simulink model "ProyectoAutomatasSimulink_jona"  (R2017a)
settings: Solver=FixedStepAuto  StartTime=0.0  StopTime=inf  FixedStep=dt  RelTol=1e-3
values from neighbouring files (symbols this model uses):
  amaxh = 1    [ProyectoAutomatas.m]
  amaxt = 1    [ProyectoAutomatas.m]
  bah = Jh*nh*wposh    (= 1200355.55556)    [ProyectoAutomatas.m]
  bat = Jt*nt*wpost    (= 1966933.33333)    [ProyectoAutomatas.m]
  bh = beqh/Rd^2    (= 32)    [ProyectoAutomatas.m]
  bt = beqc/Rw^2    (= 120)    [ProyectoAutomatas.m]
  bw = 30*10^3    (= 30000)    [ProyectoAutomatas.m]
  distanciaSegMaxCarro = geometria.xt_max-constSegCarro    [ProyectoAutomatas.m]
  distanciaSegMinCarro = geometria.xt_min+constSegCarro    [ProyectoAutomatas.m]
  dt = 0.001    [ProyectoAutomatas.m]
  g = 9.80665    [ProyectoAutomatas.m]
  Kisah = Ksah*wposh/nh    (= 150044444444)    [ProyectoAutomatas.m]
  Kisat = Ksat*wpost/nt    (= 245866666667)    [ProyectoAutomatas.m]
  Ksah = bah*wposh    (= 600177777.778)    [ProyectoAutomatas.m]
  Ksat = bat*wpost    (= 983466666.667)    [ProyectoAutomatas.m]
  Kw = 1800*10^3    (= 1800000)    [ProyectoAutomatas.m]
  l_max_cable = 65    [ProyectoAutomatas.m]
  l_min_cable = 5    [ProyectoAutomatas.m]
  lh0 = 5    [ProyectoAutomatas.m]
  longitudSegMaxCable = l_max_cable-constSegCable    (= 60)    [ProyectoAutomatas.m]
  longitudSegMinCable = l_min_cable+constSegCable    (= 10)    [ProyectoAutomatas.m]
  mc = 50000    [ProyectoAutomatas.m]
  Mh = (Jdh+Jmh*rh^2)/Rd^2    (= 48014.2222222)    [ProyectoAutomatas.m]
  ml0 = 15000    [ProyectoAutomatas.m]
  mlfull = 65000    [ProyectoAutomatas.m]
  Mt = mc+(Jwc+Jmc*rc^2)/Rw^2    (= 59008)    [ProyectoAutomatas.m]
  na = 3    [ProyectoAutomatas.m]
  ponderaPIDangulo = -1/1.3e19    (= -7.69230769231e-20)    [ProyectoAutomatas.m]
  rc = 15    [ProyectoAutomatas.m]
  Rd = 0.75    [ProyectoAutomatas.m]
  rh = 30    [ProyectoAutomatas.m]
  Rw = 0.5    [ProyectoAutomatas.m]
  tiempoTransicionAutMan = 1    [ProyectoAutomatas.m]
  vh0 = 0    [ProyectoAutomatas.m]
  vlx0 = 0    [ProyectoAutomatas.m]
  vly0 = 0    [ProyectoAutomatas.m]
  vmaxh = 3    [ProyectoAutomatas.m]
  vmaxhfull = 1.5    [ProyectoAutomatas.m]
  vmaxhSobrepeso = 0.1    [ProyectoAutomatas.m]
  vmaxt = 4    [ProyectoAutomatas.m]
  vt0 = 0    [ProyectoAutomatas.m]
  xl0 = -30    [ProyectoAutomatas.m]
  xt0 = -30    [ProyectoAutomatas.m]
  xt_max = 50    [ProyectoAutomatas.m]
  xt_max_max = 51    [ProyectoAutomatas.m]
  xt_min = -30    [ProyectoAutomatas.m]
  yl0 = yt0-lh0-ml0*g/Kw    (= 39.9182779167)    [ProyectoAutomatas.m]
  yt0 = 45    [ProyectoAutomatas.m]
undefined symbols (not defined in the file or in its folder): geometria
libraries: vrlib x1
settings Model: Creator=Garcia Obredor  LastModifiedBy=yellow submarine
settings DataIOCC: LimitDataPoints=on  SaveFormat=Array  SignalLoggingSaveFormat=ModelDataLogs
settings OptimizationCC: BlockReduction=off  BooleanDataType=off  LifeSpan=inf
settings DebuggingCC: SaveWithParameterizedLinksMsg=none  UnderspecifiedInitializationDetection=Classic  MergeDetectMultiDrivingBlocksExec=none  SignalResolutionControl=TryResolveAllWithWarning  MultiTaskDSMMsg=warning  MultiTaskCondExecSysMsg=none  SFUnexpectedBacktrackingDiag=warning  SFNoUnconditionalDefaultTransitionDiag=warning  SFExecutionAtInitializationDiag=none
settings HardwareCC: ProdBitPerPointer=32  ProdBitPerSizeT=32  ProdBitPerPtrDiffT=32  ProdLargestAtomicFloat=None  ProdIntDivRoundTo=Undefined  ProdEndianess=Unspecified  ProdWordSize=32  ProdHWDeviceType=32-bit Generic  TargetBitPerPointer=64  TargetBitPerSizeT=64  TargetBitPerPtrDiffT=64  TargetLongLongMode=on  TargetIntDivRoundTo=Zero  TargetEndianess=LittleEndian  TargetWordSize=64  TargetHWDeviceType=MATLAB Host  ProdEqTarget=off
settings ModelReferenceCC: PropagateSignalLabelsOutOfModel=off
settings GRTTargetCC: TargetLangStandard=C89/C90 (ANSI)  GeneratePreprocessorConditionals=Disable all
settings ConfigComp: CovMetricSettings=dw  CovHtmlReporting=on  CovSaveCumulativeToWorkspaceVar=on  CovSaveSingleToWorkspaceVar=on  CovExternalEMLEnable=off

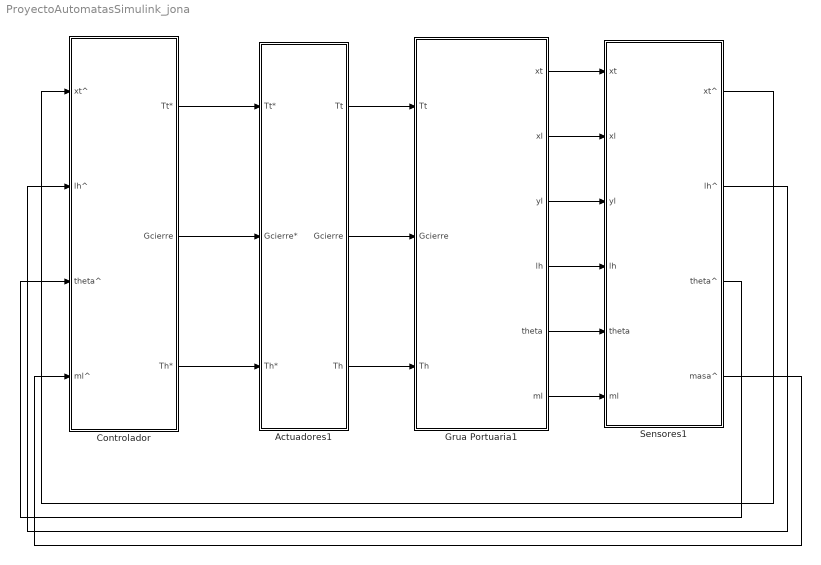
== system ProyectoAutomatasSimulink_jona ==
  Actuadores1 : Subsystem
  Controlador : Subsystem
  Grua Portuaria1 : Subsystem
  Sensores1 : Subsystem
  wires:
  Controlador/2(Gcierre) -> Actuadores1/2(Gcierre*)
  Grua Portuaria1/6(ml) -> Sensores1/6(ml)
  Grua Portuaria1/1(xt) -> Sensores1/1(xt)
  Actuadores1/2(Gcierre) -> Grua Portuaria1/2(Gcierre)
  Grua Portuaria1/5(theta) -> Sensores1/5(theta)
  Controlador/3(Th*) -> Actuadores1/3(Th*)
  Actuadores1/3(Th) -> Grua Portuaria1/3(Th)
  Actuadores1/1(Tt) -> Grua Portuaria1/1(Tt)
  Grua Portuaria1/3(yl) -> Sensores1/3(yl)
  Grua Portuaria1/4(lh) -> Sensores1/4(lh)
  Controlador/1(Tt*) -> Actuadores1/1(Tt*)
  Grua Portuaria1/2(xl) -> Sensores1/2(xl)
  Sensores1/1(xt^) -> Controlador/1(xt^)
  Sensores1/2(lh^) -> Controlador/2(lh^)
  Sensores1/3(theta^) -> Controlador/3(theta^)
  Sensores1/4(masa^) -> Controlador/4(ml^)

== system ProyectoAutomatasSimulink_jona/Actuadores1 ==
  Tt* : Inport
  Gcierre* : Inport  Port=2
  Th* : Inport  Port=3
  Tt : Outport
  Gcierre : Outport  Port=2
  Th : Outport  Port=3
  wires:
  Tt*/1 -> Tt/1  "Tt"
  Th*/1 -> Th/1  "Th"
  Gcierre*/1 -> Gcierre/1

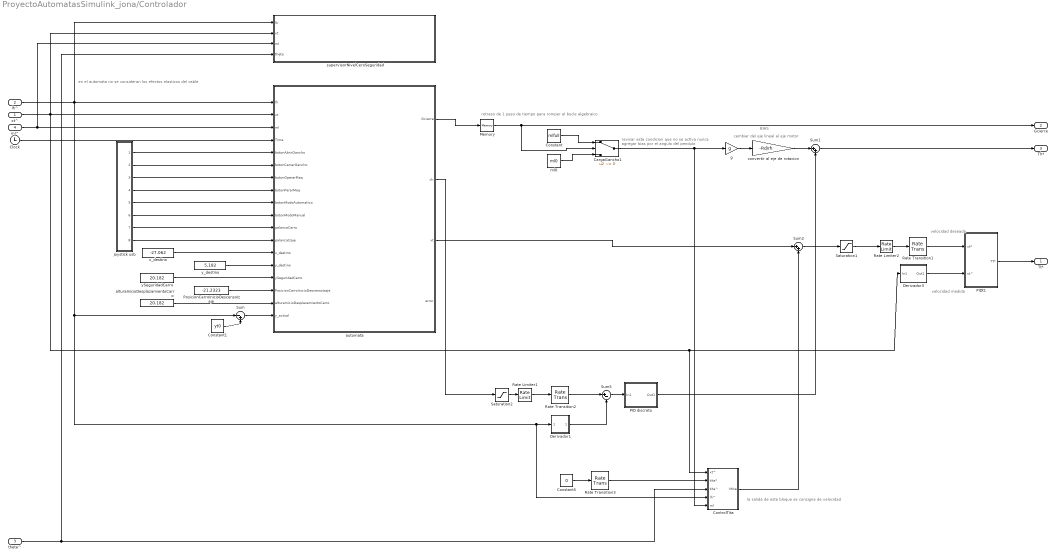
== system ProyectoAutomatasSimulink_jona/Controlador ==
  note: la salida de este bloque es consigna de velocidad
  note: cambiar del eje lineal al eje motor
  note: revisar esta condicion que no se activa nunca
      | agregar bias por el angulo del pendulo
  note: BIAS
  note: velocidad medida
  note: velocidad deseada
  note: retraso de 1 paso de tiempo para romper el bucle algebraico
  note: en el automata no se consideran los efectos elasticos del cable
  xt^ : Inport
  lh^ : Inport  Port=2
  theta^ : Inport  Port=3
  ml^ : Inport  Port=4
  CargaGancho1 : Switch  Criteria=u2 ~= 0  Threshold=0.5
  Clock : Clock
  Constant : Constant  Value=mlfull
  Constant1 : Constant  Value=yt0
  Constant5 : Constant  Value=0
  ControlTita : Subsystem
  Derivador1 : Subsystem
  Derivador3 : Subsystem
  Memory : Memory
  PID discreto : Subsystem
  PIDt1 : Subsystem
  PosicionCarroInicioDescensoIzaje : Constant  Value=-21.2323
  Rate Limiter1 : RateLimiter  RisingSlewLimit=amaxh  FallingSlewLimit=-amaxh  SampleTimeMode=inherited
  Rate Limiter2 : RateLimiter  RisingSlewLimit=amaxt  FallingSlewLimit=-amaxt  SampleTimeMode=inherited
  Rate Transition1 : RateTransition  OutPortSampleTime=dt
  Rate Transition2 : RateTransition  X0=5  OutPortSampleTime=dt
  Rate Transition3 : RateTransition  OutPortSampleTime=dt
  Saturation1 : Saturate  UpperLimit=vmaxt  LowerLimit=-vmaxt
  Saturation2 : Saturate  UpperLimit=vmaxh  LowerLimit=-vmaxh
  Sum : Sum  Inputs=|-+
  Sum1 : Sum  Inputs=|++
  Sum2 : Sum  Inputs=|++
  Sum5 : Sum  Inputs=|+-
  alturaInicioDesplazamientoCarro : Constant  Value=20.182
  automata : Stateflow chart  TreatAsAtomicUnit=on
  convertir al eje de rotacion : Gain  Gain=-Rd/rh
  g : Gain  Gain=g
  joystick usb : Subsystem
  "ml0 " : Constant  Value=ml0
  supervisorNivelCeroSeguridad : Stateflow chart  TreatAsAtomicUnit=on
  x_destino : Constant  Value=-27.062
  ySeguridadCarro : Constant  Value=20.182
  y_destino : Constant  Value=5.182
  Tt* : Outport
  Gcierre : Outport  Port=2
  Th* : Outport  Port=3
  wires:
  ml^/1 -> automata/3(ml), supervisorNivelCeroSeguridad/3(ml)
  automata/2(vh) -> Saturation2/1
  joystick usb/7(Out8) -> automata/11(palancaCarro)
  joystick usb/1(Out1) -> automata/5(botonAbrirGancho)
  joystick usb/2(Out2) -> automata/6(botonCerrarGancho)
  joystick usb/8(Out9) -> automata/12(palancaIzaje)
  joystick usb/4(Out4) -> automata/8(botonPararMaq)
  joystick usb/5(Out6) -> automata/9(botonModoAutomatico)
  joystick usb/6(Out7) -> automata/10(botonModoManual)
  joystick usb/3(Out3) -> automata/7(botonOperarMaq)
  Saturation1/1 -> Rate Limiter2/1
  Rate Transition1/1 -> PIDt1/1(xt*)
  Rate Limiter2/1 -> Rate Transition1/1
  Derivador3/1(Out1) -> PIDt1/2(xt^)
  xt^/1 -> supervisorNivelCeroSeguridad/2(xt), automata/2(xt), Derivador3/1(In1), ControlTita/1(xt^)
  Sum1/1 -> Th*/1
  automata/1(Gcierre) -> Memory/1
  "ml0 "/1 -> CargaGancho1/3
  Constant/1 -> CargaGancho1/1
  Memory/1 -> CargaGancho1/2, Gcierre/1
  PIDt1/1(Tt*) -> Tt*/1
  g/1 -> convertir al eje de rotacion/1
  convertir al eje de rotacion/1 -> Sum1/1
  PID discreto/1(Out1) -> Sum1/2
  Rate Transition2/1 -> Sum5/1
  Sum5/1 -> PID discreto/1(In1)
  Rate Limiter1/1 -> Rate Transition2/1
  Saturation2/1 -> Rate Limiter1/1
  Derivador1/1(Out1) -> Sum5/2
  automata/3(vt) -> Sum2/1
  Constant5/1 -> Rate Transition3/1
  Rate Transition3/1 -> ControlTita/2(tita*)
  lh^/1 -> supervisorNivelCeroSeguridad/1(lh), automata/1(lh), ControlTita/4(lh^), Derivador1/1(In1), Sum/1
  theta^/1 -> ControlTita/3(tita^), supervisorNivelCeroSeguridad/4(theta)
  CargaGancho1/1 -> ControlTita/5(ml), g/1
  ySeguridadCarro/1 -> automata/15(ySeguridadCarro)
  PosicionCarroInicioDescensoIzaje/1 -> automata/16(PosicionCarroInicioDescensoIzaje)
  alturaInicioDesplazamientoCarro/1 -> automata/17(alturaInicioDesplazamientoCarro)
  x_destino/1 -> automata/13(x_destino)
  Constant1/1 -> Sum/2
  Sum/1 -> automata/18(y_actual)
  y_destino/1 -> automata/14(y_destino)
  Sum2/1 -> Saturation1/1
  ControlTita/1(Vtita) -> Sum2/2
  Clock/1 -> automata/4(Time)

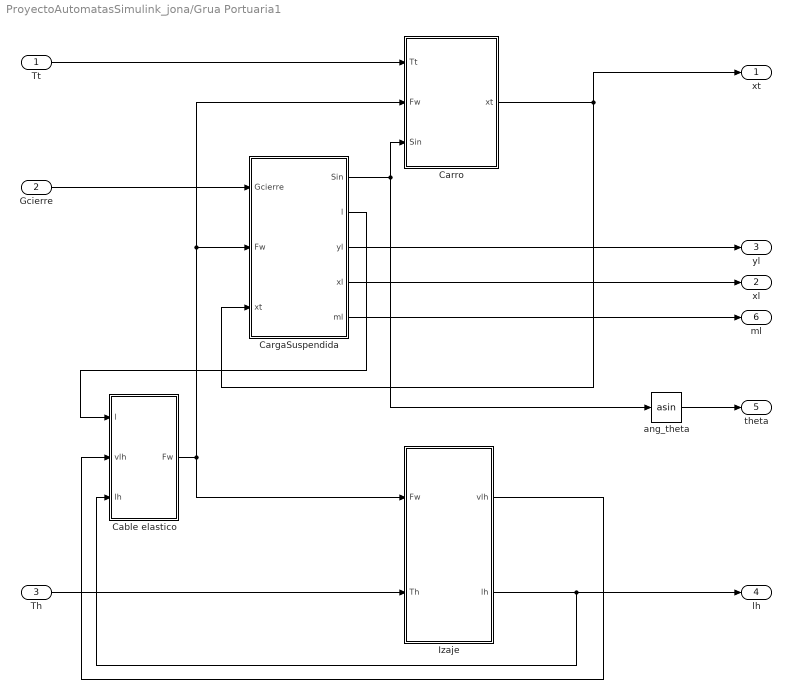
== system ProyectoAutomatasSimulink_jona/Grua Portuaria1 ==
  Tt : Inport
  Gcierre : Inport  Port=2
  Th : Inport  Port=3
  Cable elastico : Subsystem
  CargaSuspendida : Subsystem
  Carro : Subsystem
  Izaje : Subsystem
  ang_theta : Trigonometry  Operator=asin
  xt : Outport
  xl : Outport  Port=2
  yl : Outport  Port=3
  lh : Outport  Port=4
  theta : Outport  Port=5
  ml : Outport  Port=6
  wires:
  Izaje/1(vlh) -> Cable elastico/2(vlh)
  CargaSuspendida/1(Sin) -> Carro/3(Sin), ang_theta/1
  Th/1 -> Izaje/2(Th)
  Izaje/2(lh) -> Cable elastico/3(lh), lh/1
  Carro/1(xt) -> xt/1, CargaSuspendida/3(xt)
  Gcierre/1 -> CargaSuspendida/1(Gcierre)
  Tt/1 -> Carro/1(Tt)
  CargaSuspendida/2(l) -> Cable elastico/1(l)
  Cable elastico/1(Fw) -> Izaje/1(Fw), Carro/2(Fw), CargaSuspendida/2(Fw)
  ang_theta/1 -> theta/1
  CargaSuspendida/5(ml) -> ml/1
  CargaSuspendida/4(xl) -> xl/1
  CargaSuspendida/3(yl) -> yl/1

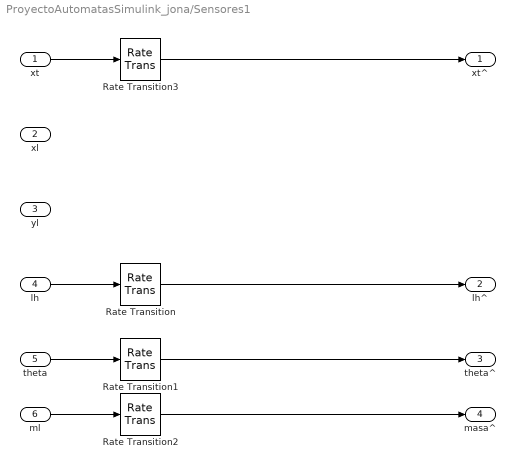
== system ProyectoAutomatasSimulink_jona/Sensores1 ==
  xt : Inport
  xl : Inport  Port=2
  yl : Inport  Port=3
  lh : Inport  Port=4
  theta : Inport  Port=5
  ml : Inport  Port=6
  Rate Transition : RateTransition  X0=5  OutPortSampleTime=dt
  Rate Transition1 : RateTransition  OutPortSampleTime=dt
  Rate Transition2 : RateTransition  X0=ml0  OutPortSampleTime=dt
  Rate Transition3 : RateTransition  X0=-30  OutPortSampleTime=dt
  xt^ : Outport
  lh^ : Outport  Port=2
  theta^ : Outport  Port=3
  masa^ : Outport  Port=4
  wires:
  theta/1 -> Rate Transition1/1
  xt/1 -> Rate Transition3/1
  Rate Transition1/1 -> theta^/1
  ml/1 -> Rate Transition2/1
  lh/1 -> Rate Transition/1
  Rate Transition/1 -> lh^/1
  Rate Transition3/1 -> xt^/1
  Rate Transition2/1 -> masa^/1

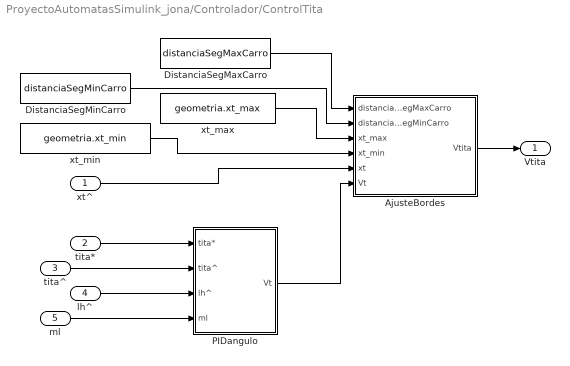
== system ProyectoAutomatasSimulink_jona/Controlador/ControlTita ==
  xt^ : Inport
  tita* : Inport  Port=2
  tita^ : Inport  Port=3
  lh^ : Inport  Port=4
  ml : Inport  Port=5
  AjusteBordes : MATLAB Function  TreatAsAtomicUnit=on
  DistanciaSegMaxCarro : Constant  Value=distanciaSegMaxCarro
  DistanciaSegMinCarro : Constant  Value=distanciaSegMinCarro
  PIDangulo : Subsystem
  xt_max : Constant  Value=geometria.xt_max
  xt_min : Constant  Value=geometria.xt_min
  Vtita : Outport
  wires:
  tita*/1 -> PIDangulo/1(tita*)
  ml/1 -> PIDangulo/4(ml)
  lh^/1 -> PIDangulo/3(lh^)
  AjusteBordes/1(Vtita) -> Vtita/1
  tita^/1 -> PIDangulo/2(tita^)
  PIDangulo/1(Vt) -> AjusteBordes/6(Vt)
  xt^/1 -> AjusteBordes/5(xt)
  DistanciaSegMaxCarro/1 -> AjusteBordes/1(distanciaSegMaxCarro)
  DistanciaSegMinCarro/1 -> AjusteBordes/2(distanciaSegMinCarro)
  xt_max/1 -> AjusteBordes/3(xt_max)
  xt_min/1 -> AjusteBordes/4(xt_min)

== system ProyectoAutomatasSimulink_jona/Controlador/Derivador1 ==
  In1 : Inport
  1/dt : Gain  Gain=1/dt
  Delay3 : Delay  DelayLength=1  InitialCondition=5  SampleTime=dt
  Sum6 : Sum  Inputs=|+-
  Out1 : Outport
  wires:
  In1/1 -> Delay3/1, Sum6/1
  Delay3/1 -> Sum6/2
  Sum6/1 -> 1/dt/1
  1/dt/1 -> Out1/1

== system ProyectoAutomatasSimulink_jona/Controlador/Derivador3 ==
  In1 : Inport
  1/dt : Gain  Gain=1/dt
  Delay3 : Delay  DelayLength=1  InitialCondition=-30  SampleTime=dt
  Sum6 : Sum  Inputs=|+-
  Out1 : Outport
  wires:
  In1/1 -> Delay3/1, Sum6/1
  Delay3/1 -> Sum6/2
  Sum6/1 -> 1/dt/1
  1/dt/1 -> Out1/1

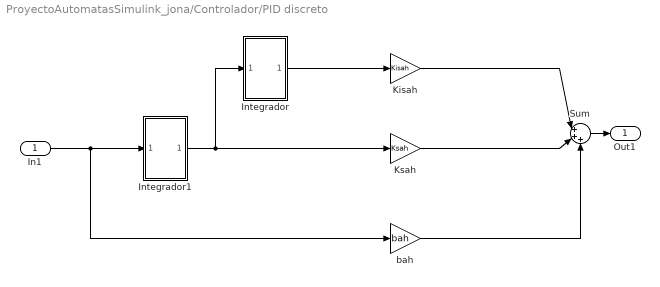
== system ProyectoAutomatasSimulink_jona/Controlador/PID discreto ==
  In1 : Inport
  Integrador : Subsystem
  Integrador1 : Subsystem
  Kisah : Gain  Gain=Kisah
  Ksah : Gain  Gain=Ksah
  Sum : Sum  Inputs=|+++
  bah : Gain  Gain=bah
  Out1 : Outport
  wires:
  In1/1 -> Integrador1/1(In1), bah/1
  bah/1 -> Sum/3
  Sum/1 -> Out1/1
  Ksah/1 -> Sum/2
  Kisah/1 -> Sum/1
  Integrador/1(Out1) -> Kisah/1
  Integrador1/1(Out1) -> Integrador/1(In1), Ksah/1

== system ProyectoAutomatasSimulink_jona/Controlador/PIDt1 ==
  xt* : Inport
  xt^ : Inport  Port=2
  PID discreto : Subsystem
  Scope : Scope
  Sum5 : Sum  Inputs=|+-
  Tt* : Outport
  wires:
  xt*/1 -> Sum5/1
  xt^/1 -> Sum5/2
  Sum5/1 -> Scope/1, PID discreto/1(In1)
  PID discreto/1(Out1) -> Tt*/1

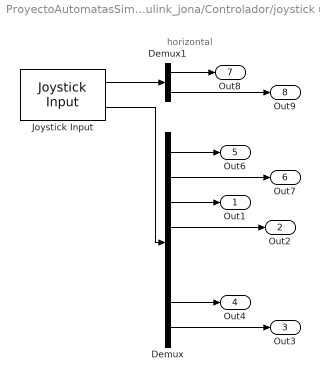
== system ProyectoAutomatasSimulink_jona/Controlador/joystick usb ==
  note: horizontal
  Demux : Demux  Outputs=8
  Demux1 : Demux  Outputs=2
  Joystick Input : vrlib/Joystick Input  joyid=1  adjustports=on  forcefeed=off
      settings: SourceProductBaseCode=VR
  Out1 : Outport
  Out2 : Outport  Port=2
  Out3 : Outport  Port=3
  Out4 : Outport  Port=4
  Out6 : Outport  Port=5
  Out7 : Outport  Port=6
  Out8 : Outport  Port=7
  Out9 : Outport  Port=8
  wires:
  Demux/8 -> Out3/1
  Demux/1 -> Out6/1
  Joystick Input/2 -> Demux/1
  Demux/2 -> Out7/1
  Joystick Input/1 -> Demux1/1
  Demux/7 -> Out4/1
  Demux1/1 -> Out8/1
  Demux1/2 -> Out9/1
  Demux/4 -> Out2/1
  Demux/3 -> Out1/1

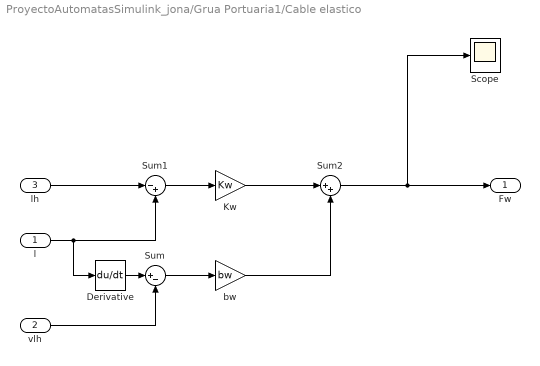
== system ProyectoAutomatasSimulink_jona/Grua Portuaria1/Cable elastico ==
  l : Inport
  vlh : Inport  Port=2
  lh : Inport  Port=3
  Derivative : Derivative
  Kw : Gain  Gain=Kw
  Scope : Scope
  Sum : Sum  Inputs=|+-
  Sum1 : Sum  Inputs=|-+
  Sum2 : Sum  Inputs=|++
  bw : Gain  Gain=bw
  Fw : Outport
  wires:
  l/1 -> Derivative/1, Sum1/2
  Derivative/1 -> Sum/1
  vlh/1 -> Sum/2
  Sum1/1 -> Kw/1
  Sum/1 -> bw/1
  Kw/1 -> Sum2/1
  bw/1 -> Sum2/2
  Sum2/1 -> Scope/1, Fw/1
  lh/1 -> Sum1/1

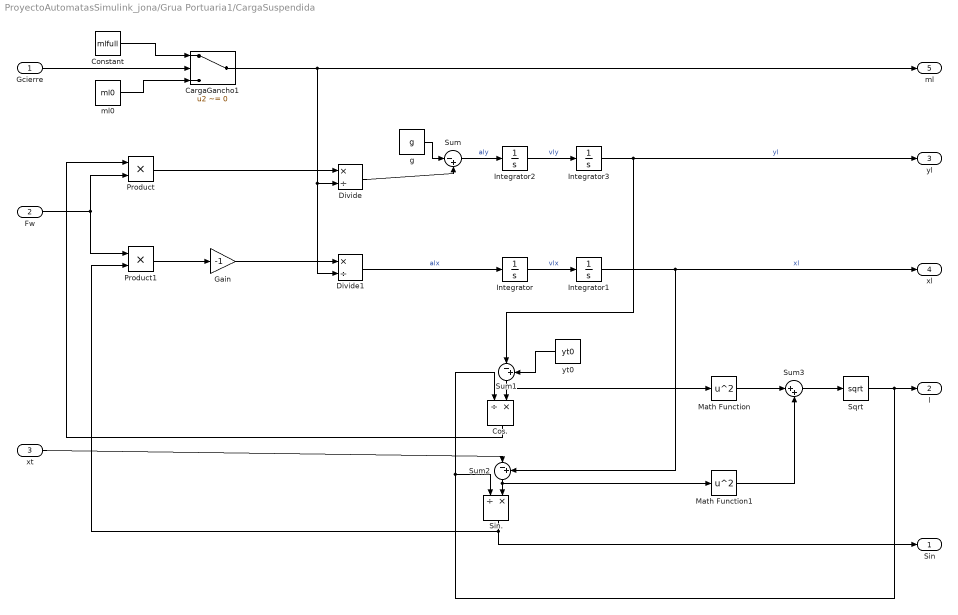
== system ProyectoAutomatasSimulink_jona/Grua Portuaria1/CargaSuspendida ==
  Gcierre : Inport
  Fw : Inport  Port=2
  xt : Inport  Port=3
  CargaGancho1 : Switch  Criteria=u2 ~= 0  Threshold=0.5
  Constant : Constant  Value=mlfull
  Cos. : Product  Inputs=/*
  Divide : Product  Inputs=*/
  Divide1 : Product  Inputs=*/
  Gain : Gain  Gain=-1
  Integrator : Integrator  InitialCondition=vlx0
  Integrator1 : Integrator  InitialCondition=xl0
  Integrator2 : Integrator  InitialCondition=vly0
  Integrator3 : Integrator  InitialCondition=yl0
  Math Function : Math  Operator=square  SaturateOnIntegerOverflow=on
  Math Function1 : Math  Operator=square  SaturateOnIntegerOverflow=on
  Product : Product
  Product1 : Product
  Sin. : Product  Inputs=/*
  Sqrt : Sqrt  SaturateOnIntegerOverflow=on
  Sum : Sum  Inputs=|-+
  Sum1 : Sum  Inputs=|-+
  Sum2 : Sum  Inputs=|-+
  Sum3 : Sum  Inputs=|++
  g : Constant  Value=g
  "ml0 " : Constant  Value=ml0
  yt0 : Constant  Value=yt0
  Sin : Outport
  l : Outport  Port=2
  yl : Outport  Port=3
  xl : Outport  Port=4
  ml : Outport  Port=5
  wires:
  CargaGancho1/1 -> ml/1, Divide/2, Divide1/2
  Gcierre/1 -> CargaGancho1/2
  Fw/1 -> Product1/1, Product/2
  Product/1 -> Divide/1
  Product1/1 -> Gain/1
  Gain/1 -> Divide1/1
  Divide/1 -> Sum/2
  g/1 -> Sum/1
  Integrator/1 -> Integrator1/1  "vlx"
  Integrator1/1 -> xl/1, Sum2/2  "xl"
  Integrator2/1 -> Integrator3/1  "vly"
  Sum1/1 -> Cos./2, Math Function/1
  yt0/1 -> Sum1/2
  Integrator3/1 -> Sum1/1, yl/1  "yl"
  Cos./1 -> Product/1
  Sum2/1 -> Math Function1/1, Sin./2
  xt/1 -> Sum2/1
  Sin./1 -> Sin/1, Product1/2
  Math Function/1 -> Sum3/1
  Math Function1/1 -> Sum3/2
  Sum3/1 -> Sqrt/1
  Constant/1 -> CargaGancho1/1
  "ml0 "/1 -> CargaGancho1/3
  Sqrt/1 -> Cos./1, Sin./1, l/1
  Sum/1 -> Integrator2/1  "aly"
  Divide1/1 -> Integrator/1  "alx"

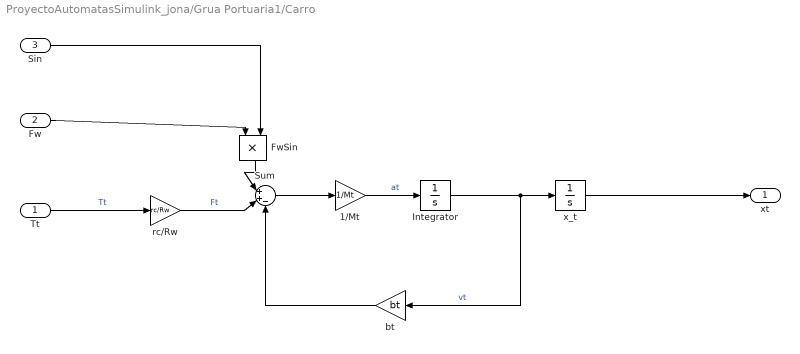
== system ProyectoAutomatasSimulink_jona/Grua Portuaria1/Carro ==
  Tt : Inport
  Fw : Inport  Port=2
  Sin : Inport  Port=3
  1/Mt : Gain  Gain=1/Mt
  FwSin : Product
  Integrator : Integrator  InitialCondition=vt0
  Sum : Sum  Inputs=|++-
  bt : Gain  Gain=bt
  rc/Rw : Gain  Gain=rc/Rw
  x_t : Integrator  InitialCondition=xt0
  xt : Outport
  wires:
  x_t/1 -> xt/1
  rc/Rw/1 -> Sum/2  "Ft"
  Tt/1 -> rc/Rw/1  "Tt"
  1/Mt/1 -> Integrator/1  "at"
  bt/1 -> Sum/3
  Sum/1 -> 1/Mt/1
  Integrator/1 -> bt/1, x_t/1  "vt"
  Sin/1 -> FwSin/2
  FwSin/1 -> Sum/1
  Fw/1 -> FwSin/1

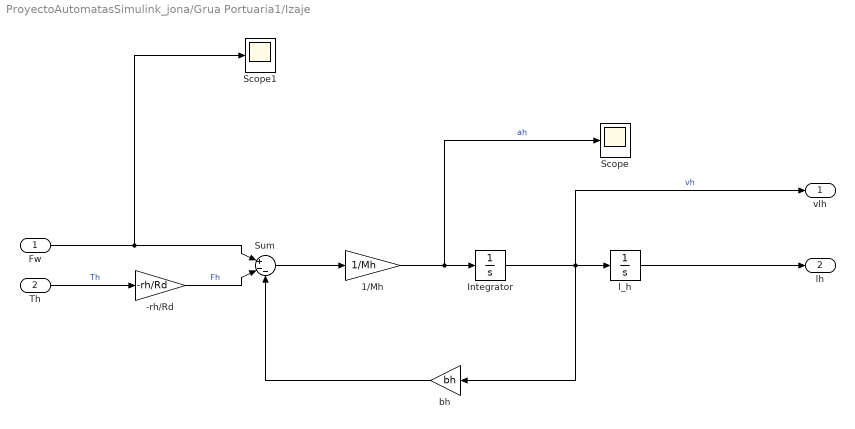
== system ProyectoAutomatasSimulink_jona/Grua Portuaria1/Izaje ==
  Fw : Inport
  Th : Inport  Port=2
  "-rh/Rd\t" : Gain  Gain=-rh/Rd
  1/Mh : Gain  Gain=1/Mh
  Integrator : Integrator  InitialCondition=vh0
  Scope : Scope
  Scope1 : Scope
  Sum : Sum  Inputs=|+--
  bh : Gain  Gain=bh
  l_h : Integrator  InitialCondition=lh0
  vlh : Outport
  lh : Outport  Port=2
  wires:
  l_h/1 -> lh/1
  "-rh/Rd\t"/1 -> Sum/2  "Fh"
  Th/1 -> "-rh/Rd\t"/1  "Th"
  1/Mh/1 -> Scope/1, Integrator/1  "ah"
  bh/1 -> Sum/3
  Sum/1 -> 1/Mh/1
  Integrator/1 -> vlh/1, bh/1, l_h/1  "vh"
  Fw/1 -> Scope1/1, Sum/1

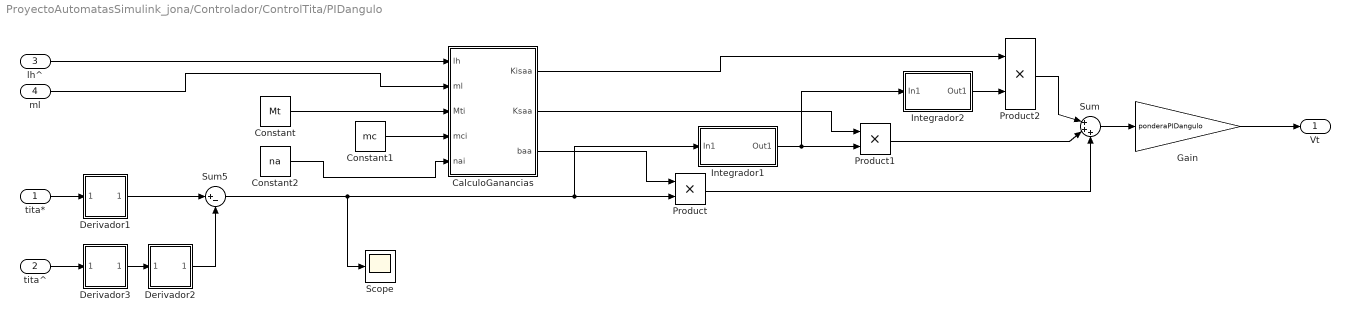
== system ProyectoAutomatasSimulink_jona/Controlador/ControlTita/PIDangulo ==
  tita* : Inport
  tita^ : Inport  Port=2
  lh^ : Inport  Port=3
  ml : Inport  Port=4
  CalculoGanancias : MATLAB Function  TreatAsAtomicUnit=on
  Constant : Constant  Value=Mt
  Constant1 : Constant  Value=mc
  Constant2 : Constant  Value=na
  Derivador1 : Subsystem
  Derivador2 : Subsystem
  Derivador3 : Subsystem
  Gain : Gain  Gain=ponderaPIDangulo
  Integrador1 : Subsystem
  Integrador2 : Subsystem
  Product : Product
  Product1 : Product
  Product2 : Product
  Scope : Scope
  Sum : Sum  Inputs=|+++
  Sum5 : Sum  Inputs=|+-
  Vt : Outport
  wires:
  tita*/1 -> Derivador1/1(In1)
  lh^/1 -> CalculoGanancias/1(lh)
  Sum/1 -> Gain/1
  Product/1 -> Sum/3
  Integrador1/1(Out1) -> Integrador2/1(In1), Product1/2
  Product1/1 -> Sum/2
  Integrador2/1(Out1) -> Product2/2
  tita^/1 -> Derivador3/1(In1)
  Sum5/1 -> Scope/1, Integrador1/1(In1), Product/2
  CalculoGanancias/3(baa) -> Product/1
  CalculoGanancias/2(Ksaa) -> Product1/1
  CalculoGanancias/1(Kisaa) -> Product2/1
  ml/1 -> CalculoGanancias/2(ml)
  Constant/1 -> CalculoGanancias/3(Mti)
  Constant1/1 -> CalculoGanancias/4(mci)
  Constant2/1 -> CalculoGanancias/5(nai)
  Derivador3/1(Out1) -> Derivador2/1(In1)
  Derivador1/1(Out1) -> Sum5/1
  Gain/1 -> Vt/1
  Product2/1 -> Sum/1
  Derivador2/1(Out1) -> Sum5/2

== system ProyectoAutomatasSimulink_jona/Controlador/PID discreto/Integrador ==
  In1 : Inport
  Delay3 : Delay  DelayLength=1  SampleTime=dt
  Sum6 : Sum  Inputs=|++
  dt : Gain  Gain=dt
  Out1 : Outport
  wires:
  Delay3/1 -> Sum6/2
  Sum6/1 -> Out1/1, Delay3/1
  dt/1 -> Sum6/1
  In1/1 -> dt/1

== system ProyectoAutomatasSimulink_jona/Controlador/PID discreto/Integrador1 ==
  In1 : Inport
  Delay3 : Delay  DelayLength=1  SampleTime=dt
  Sum6 : Sum  Inputs=|++
  dt : Gain  Gain=dt
  Out1 : Outport
  wires:
  Delay3/1 -> Sum6/2
  Sum6/1 -> Out1/1, Delay3/1
  dt/1 -> Sum6/1
  In1/1 -> dt/1

== system ProyectoAutomatasSimulink_jona/Controlador/PIDt1/PID discreto ==
  In1 : Inport
  Integrador : Subsystem
  Integrador1 : Subsystem
  Kisat : Gain  Gain=Kisat
  Ksat : Gain  Gain=Ksat
  Sum : Sum  Inputs=|+++
  bat : Gain  Gain=bat
  Out1 : Outport
  wires:
  bat/1 -> Sum/3
  Ksat/1 -> Sum/2
  Kisat/1 -> Sum/1
  Sum/1 -> Out1/1
  In1/1 -> Integrador1/1(In1), bat/1
  Integrador/1(Out1) -> Kisat/1
  Integrador1/1(Out1) -> Integrador/1(In1), Ksat/1

== system ProyectoAutomatasSimulink_jona/Controlador/ControlTita/PIDangulo/Derivador1 ==
  In1 : Inport
  1/dt : Gain  Gain=1/dt
  Delay3 : Delay  DelayLength=1  InitialCondition=0  SampleTime=dt
  Sum6 : Sum  Inputs=|+-
  Out1 : Outport
  wires:
  In1/1 -> Delay3/1, Sum6/1
  Delay3/1 -> Sum6/2
  Sum6/1 -> 1/dt/1
  1/dt/1 -> Out1/1

== system ProyectoAutomatasSimulink_jona/Controlador/ControlTita/PIDangulo/Derivador2 ==
  In1 : Inport
  1/dt : Gain  Gain=1/dt
  Delay3 : Delay  DelayLength=1  InitialCondition=0  SampleTime=dt
  Sum6 : Sum  Inputs=|+-
  Out1 : Outport
  wires:
  In1/1 -> Delay3/1, Sum6/1
  Delay3/1 -> Sum6/2
  Sum6/1 -> 1/dt/1
  1/dt/1 -> Out1/1

== system ProyectoAutomatasSimulink_jona/Controlador/ControlTita/PIDangulo/Derivador3 ==
  In1 : Inport
  1/dt : Gain  Gain=1/dt
  Delay3 : Delay  DelayLength=1  InitialCondition=0  SampleTime=dt
  Sum6 : Sum  Inputs=|+-
  Out1 : Outport
  wires:
  In1/1 -> Delay3/1, Sum6/1
  Delay3/1 -> Sum6/2
  Sum6/1 -> 1/dt/1
  1/dt/1 -> Out1/1

== system ProyectoAutomatasSimulink_jona/Controlador/ControlTita/PIDangulo/Integrador1 ==
  In1 : Inport
  Delay3 : Delay  DelayLength=1  SampleTime=dt
  Sum6 : Sum  Inputs=|++
  dt : Gain  Gain=dt
  Out1 : Outport
  wires:
  Delay3/1 -> Sum6/2
  Sum6/1 -> Out1/1, Delay3/1
  dt/1 -> Sum6/1
  In1/1 -> dt/1

== system ProyectoAutomatasSimulink_jona/Controlador/ControlTita/PIDangulo/Integrador2 ==
  In1 : Inport
  Delay3 : Delay  DelayLength=1  SampleTime=dt
  Sum6 : Sum  Inputs=|++
  dt : Gain  Gain=dt
  Out1 : Outport
  wires:
  Delay3/1 -> Sum6/2
  Sum6/1 -> Out1/1, Delay3/1
  dt/1 -> Sum6/1
  In1/1 -> dt/1

== system ProyectoAutomatasSimulink_jona/Controlador/PIDt1/PID discreto/Integrador ==
  In1 : Inport
  Delay3 : Delay  DelayLength=1  SampleTime=dt
  Sum6 : Sum  Inputs=|++
  dt : Gain  Gain=dt
  Out1 : Outport
  wires:
  Delay3/1 -> Sum6/2
  Sum6/1 -> Out1/1, Delay3/1
  dt/1 -> Sum6/1
  In1/1 -> dt/1

== system ProyectoAutomatasSimulink_jona/Controlador/PIDt1/PID discreto/Integrador1 ==
  In1 : Inport
  Delay3 : Delay  DelayLength=1  SampleTime=dt
  Sum6 : Sum  Inputs=|++
  dt : Gain  Gain=dt
  Out1 : Outport
  wires:
  Delay3/1 -> Sum6/2
  Sum6/1 -> Out1/1, Delay3/1
  dt/1 -> Sum6/1
  In1/1 -> dt/1

== stateflow chart ProyectoAutomatasSimulink_jona/Controlador/supervisorNivelCeroSeguridad ==
  state normal
  state fallaLimites
  (default) -> normal
  normal -> fallaLimites : [xt>xt_max_max]
  data: lh input; xt input; ml input; theta input; geometria parameter; xt_max_max parameter

== stateflow chart ProyectoAutomatasSimulink_jona/Controlador/automata ==
  state automata
    state tableroDeControl [parallel]
      settings: executionOrder=1
      state tableroInactivo
      state tableroActivo
        entry: tiempoTableroActivo = temporalCount(sec);
        during: tiempoTableroActivo = temporalCount(sec);
      (default) -> tableroInactivo
      tableroActivo -> tableroInactivo [order 1] : [tiempoTableroActivo>=1]
      tableroActivo -> tableroActivo [order 2] : [botonAbrirGancho || botonCerrarGancho || botonOperarMaq || botonPararMaq || botonModoAutomatico || botonModoManual || palancaCarro~=0 || palancaIzaje~=0]
      tableroInactivo -> tableroActivo : [botonAbrirGancho || botonCerrarGancho || botonOperarMaq || botonPararMaq || botonModoAutomatico || botonModoManual || palancaCarro~=0 || palancaIzaje~=0]
    state grua [parallel]
      settings: executionOrder=2
      state espera
        entry:
        vt=0;
        vh=0;
        vtPermitida=[0  0];
        vhPermitida=[0 0];
        error=0;
      state maquinaOperando1
        note: verificar que el operario solto la palanca y sino volver al modo manual
            |  || in(tableroDeControl,tableroActivo)
        state modoDeOperacion [parallel]
          settings: executionOrder=3
          state opManual [parallel]
            settings: executionOrder=1
            state Carro [parallel]
              during:
              if palancaCarro==-1  %izquierda
              vtmanual=-vtPermitida(1); %primer valor es la permitida a la izq
              elseif palancaCarro==0
              vtmanual=0;
              elseif palancaCarro==1
              vtmanual=vtPermitida(2); %segundo valor es la permitida a la der
              end
              settings: executionOrder=2
            state Izaje [parallel]
              during:
              if palancaIzaje==1  % boton hacia abajo
              vhmanual=vhPermitida(1);
              elseif palancaIzaje==0
              vhmanual=0;
              elseif palancaIzaje==-1
              vhmanual=-vhPermitida(2);
              end
              settings: executionOrder=1
          state CalculoSalidas [parallel]
            settings: executionOrder=2
            state Manual
              during:
              vt=vtmanual;
              vh=vhmanual;
            state ManualAuto
              entry: time0=Time;
              dt=0;
              during:
              dt=Time-time0;
              [vt,vh]=Transferencia(1,dt,vtmanual,vtauto,vhmanual,vhauto);
            state Automatico
              during:
              vt=vtauto;
              vh=vhauto;
            state AutoManual
              entry: time0=Time;
              dt=0;
              during:
              dt=Time-time0;
              [vt,vh]=Transferencia(-1,dt,vtmanual,vtauto,vhmanual,vhauto);
            (default) -> Manual
            Manual -> ManualAuto : [botonModoAutomatico==1]
            ManualAuto -> Automatico : [dt>=5]
            AutoManual -> Manual : [dt>=5]
            Automatico -> AutoManual [order 1] : [botonModoManual==1 || in(tableroDeControl.tableroActivo)]
            Automatico -> Manual [order 2] : [finOperacion]
          state opAutomatica1 [parallel]
            entry:
            finOperacion=0; %TODO: cambiar vt y vh para que pueda funcionar en conjunto con el control de angulo
            settings: executionOrder=3
            state start
              entry:
              finOperacion=0;
              vtauto=0;
              vhauto=0;
            state barcoAlMuelle
              state subirIzaje
                entry: vhauto=-vhPermitida(2);%-vmaxh;
              state subirYdesplazarCarro
                entry: vtauto=-vtPermitida(1);%-vmaxt;
                vhauto=-vhPermitida(2);
              state moverCarro
                entry:
                vhauto=0;
              state bajarYdesplazarCarro
                entry:
                vhauto=vmaxh;
              state bajarCarro
                entry:
                vtauto=0;
              state parar
                entry:
                %vtauto=0;
                vhauto=0;
                finOperacion=1;
              (default) -> automata.grua.maquinaOperando1.modoDeOperacion.opAutomatica1.barcoAlMuelle.subirIzaje [commented out] : [y_actual<alturaInicioDesplazamientoCarro]
              (default) -> automata.grua.maquinaOperando1.modoDeOperacion.opAutomatica1.barcoAlMuelle.subirIzaje
              automata.grua.maquinaOperando1.modoDeOperacion.opAutomatica1.barcoAlMuelle.subirIzaje -> automata.grua.maquinaOperando1.modoDeOperacion.opAutomatica1.barcoAlMuelle.subirYdesplazarCarro : [y_actual>=alturaInicioDesplazamientoCarro]
              (default) -> automata.grua.maquinaOperando1.modoDeOperacion.opAutomatica1.barcoAlMuelle.subirYdesplazarCarro [commented out] : [y_actual>ySeguridadCarro]
              automata.grua.maquinaOperando1.modoDeOperacion.opAutomatica1.barcoAlMuelle.subirYdesplazarCarro -> automata.grua.maquinaOperando1.modoDeOperacion.opAutomatica1.barcoAlMuelle.moverCarro : [y_actual>=ySeguridadCarro-0]
              automata.grua.maquinaOperando1.modoDeOperacion.opAutomatica1.barcoAlMuelle.moverCarro -> automata.grua.maquinaOperando1.modoDeOperacion.opAutomatica1.barcoAlMuelle.bajarYdesplazarCarro : [xt<PosicionCarroInicioDescensoIzaje]
              automata.grua.maquinaOperando1.modoDeOperacion.opAutomatica1.barcoAlMuelle.bajarYdesplazarCarro -> automata.grua.maquinaOperando1.modoDeOperacion.opAutomatica1.barcoAlMuelle.bajarCarro : [xt<x_destino+0]
              automata.grua.maquinaOperando1.modoDeOperacion.opAutomatica1.barcoAlMuelle.bajarCarro -> automata.grua.maquinaOperando1.modoDeOperacion.opAutomatica1.barcoAlMuelle.parar : [y_actual<=y_destino+5.5]
            state muelleAlBarco
              state subirIzaje
                entry: vhauto=-vhPermitida(2);%-vmaxh;
              state subirYdesplazarCarro
                entry: vtauto=vtPermitida(2);%vmaxt;
                vhauto=-vhPermitida(2);
              state moverCarro
                entry:
                vhauto=0;
              state bajarYdesplazarCarro
                entry:
                %vtauto=vtPermitida(2);%vmaxt;
                vhauto=vhPermitida(1);%vmaxh;
              state bajarCarro
                entry:
                vtauto=0;
                %vhauto=vhPermitida(1);%vmaxh;
              state parar
                entry:
                %vtauto=0;
                vhauto=0;
                finOperacion=1;
              (default) -> automata.grua.maquinaOperando1.modoDeOperacion.opAutomatica1.muelleAlBarco.subirIzaje [commented out] : [y_actual<ySeguridadCarro]
              (default) -> automata.grua.maquinaOperando1.modoDeOperacion.opAutomatica1.muelleAlBarco.subirIzaje
              automata.grua.maquinaOperando1.modoDeOperacion.opAutomatica1.muelleAlBarco.subirIzaje -> automata.grua.maquinaOperando1.modoDeOperacion.opAutomatica1.muelleAlBarco.subirYdesplazarCarro : [y_actual>=alturaInicioDesplazamientoCarro]
              (default) -> automata.grua.maquinaOperando1.modoDeOperacion.opAutomatica1.muelleAlBarco.subirYdesplazarCarro [commented out] : [y_actual>ySeguridadCarro]
              automata.grua.maquinaOperando1.modoDeOperacion.opAutomatica1.muelleAlBarco.subirYdesplazarCarro -> automata.grua.maquinaOperando1.modoDeOperacion.opAutomatica1.muelleAlBarco.moverCarro : [y_actual>=ySeguridadCarro-0]%ajustar la constante segun el peso del gancho
              automata.grua.maquinaOperando1.modoDeOperacion.opAutomatica1.muelleAlBarco.moverCarro -> automata.grua.maquinaOperando1.modoDeOperacion.opAutomatica1.muelleAlBarco.bajarYdesplazarCarro : [xt>=PosicionCarroInicioDescensoIzaje]
              automata.grua.maquinaOperando1.modoDeOperacion.opAutomatica1.muelleAlBarco.bajarYdesplazarCarro -> automata.grua.maquinaOperando1.modoDeOperacion.opAutomatica1.muelleAlBarco.bajarCarro : [xt>=x_destino-0]%ajustar la constante segun el peso del gancho
              automata.grua.maquinaOperando1.modoDeOperacion.opAutomatica1.muelleAlBarco.bajarCarro -> automata.grua.maquinaOperando1.modoDeOperacion.opAutomatica1.muelleAlBarco.parar : [y_actual<=y_destino+5.5]%ajustar la constante segun el peso del gancho
            (default) -> start
            start -> barcoAlMuelle [order 2] : [xt>=0 && x_destino<0]
            start -> muelleAlBarco [order 1] : [xt<0 && x_destino>=0]
            barcoAlMuelle -> start : [finOperacion]
            muelleAlBarco -> start : [finOperacion]
        state LimitesCarro [parallel]
          settings: executionOrder=2
          note: cambiar vmaxt por vPermitida?!?!?!?!?!?!?!??!?!?!?!?!??!
          state carroCercaLimiteMinimo
            during: vtPermitida(1)=rectaDosPuntos(1,0,distanciaSegMinCarro,xt_min,xt,vmaxt);
            %disp(vtPermitida(1))
          state carroDentroDeLimites
            entry: vtPermitida=[ vmaxt  vmaxt ];
            during: vtPermitida=[ vmaxt  vmaxt];
          state carroCercaLimiteMaximo
            during: vtPermitida(2)=rectaDosPuntos(1,0,distanciaSegMaxCarro,xt_max,xt,vmaxt);
            %disp(vtPermitida(2))
          (default) -> carroDentroDeLimites
          carroDentroDeLimites -> carroCercaLimiteMinimo [order 1] : [xt<=distanciaSegMinCarro]
          carroCercaLimiteMinimo -> carroDentroDeLimites : [xt>distanciaSegMinCarro]
          carroDentroDeLimites -> carroCercaLimiteMaximo [order 2] : [xt>=distanciaSegMaxCarro]
          carroCercaLimiteMaximo -> carroDentroDeLimites : [xt<distanciaSegMaxCarro]
        state supervisionIzaje [parallel]
          settings: executionOrder=1
          state limitesIzaje [parallel]
            settings: executionOrder=2
            state izajeDentroDeLimites
              entry:
              if in(gancho.Gabierto)
              vhPermitida=[vmaxh vmaxh];
              else
              vhPermitida=[vmaxhfull vmaxhfull];
              end
            state izajeCercaLimiteMaximo
              during:
              if in(gancho.Gabierto)
              vhPermitida(1)=rectaDosPuntos(vmaxh,0,longitudSegMaxCable,l_max_cable,lh);
              else
              vhPermitida(1)=rectaDosPuntos(vmaxhfull,0,longitudSegMaxCable,l_max_cable,lh);
              end
            state izajeCercaLimiteMinimo
              during:
              if in(gancho.Gabierto)
              vhPermitida(2)=rectaDosPuntos(vmaxh,0,longitudSegMinCable,l_min_cable,lh);
              else
              vhPermitida(2)=rectaDosPuntos(vmaxhfull,0,longitudSegMinCable,l_min_cable,lh);
              end
              note: el primer elemento de vhPermitida es la velocidad hacia arriba
            note: 5 metros antes del limite empieza a
                | reducir la maxima velocidad
            (default) -> izajeDentroDeLimites
            izajeCercaLimiteMaximo -> izajeDentroDeLimites : [lh<longitudSegMaxCable]
            izajeDentroDeLimites -> izajeCercaLimiteMaximo [order 1] : [lh>=longitudSegMaxCable]
            izajeDentroDeLimites -> izajeCercaLimiteMinimo [order 2] : [lh<longitudSegMinCable]
            izajeCercaLimiteMinimo -> izajeDentroDeLimites : [lh>=longitudSegMinCable]
          state gancho [parallel]
            settings: executionOrder=1
            state Gcerrado
              entry:
              Gcierre=1;
              state pesoPermitido
                entry:
                vhPermitida=[vmaxhfull vmaxhfull];
              state pesoExcedido
                entry:
                error=1;
                vhPermitida=[vmaxhSobrepeso vmaxhSobrepeso];
              (default) -> pesoPermitido
              pesoExcedido -> pesoPermitido : [ml<=mlfull]
              pesoPermitido -> pesoExcedido : [ml>mlfull]
            note: verificar que el peso suspendido este debajo del maximo!!!!!
                | la grua no opera si hay un contenedor muy pesado
            state Gabierto
              entry:
              Gcierre=0;
              vhPermitida=[vmaxh vmaxh];
            Gabierto -> Gcerrado : [botonCerrarGancho]
            Gcerrado -> Gabierto : [botonAbrirGancho]
            (default) -> Gabierto
      (default) -> espera
      maquinaOperando1 -> espera : [botonPararMaq]
      espera -> maquinaOperando1 : [botonOperarMaq]
  data: dir function_input; t function_input; Vtmanual function_input; Vtauto function_input; Vhmanual function_input; Vt function_output; Vhauto function_input; Vh function_output; y2 function_input; y1 function_input; x2 function_input; x1 function_input; x function_input; y function_output; vm function_input; y2 function_input; y1 function_input; x2 function_input; x1 function_input; x function_input; yRecta function_output; lh input; xt input; ml input; Time input; botonAbrirGancho input; botonCerrarGancho input; Gcierre output; botonOperarMaq input; botonPararMaq input; botonModoAutomatico input; botonModoManual input; palancaCarro input; palancaIzaje input; l_max_cable parameter; l_min_cable parameter; xt_min parameter; xt_max parameter; mlfull parameter; vh output; vmaxhfull parameter; vmaxh parameter; vhPermitida local; vt output; vtPermitida local; vmaxt parameter; distanciaSegMinCarro parameter; tiempoTableroActivo local; tiempoTransicionAutMan parameter; distanciaSegMaxCarro parameter; longitudSegMaxCable parameter; longitudSegMinCable parameter; error output; vmaxhSobrepeso parameter; yt0 parameter; x_destino input; y_destino input; vIzaje local; geometria parameter; ySeguridadCarro input; PosicionCarroInicioDescensoIzaje input; alturaInicioDesplazamientoCarro input; y_actual input; finOperacion local; dt local; time0 local; vhauto local; vhmanual local; vtauto local; vtmanual local
  function [Vt,Vh]  = Transferencia(dir,t,Vtmanual,Vtauto,Vhmanual,Vhauto):
    | function [Vt,Vh]  = Transferencia(dir,t,Vtmanual,Vtauto,Vhmanual,Vhauto)
    | 
    | m=1/5*dir;
    | if dir==1
    |     y1=0;
    | elseif dir==-1
    |     y1=1;
    | end
    | yRecta1=m*t+y1;
    | yRecta2=1-yRecta1;
    | Vt=yRecta1*Vtauto+yRecta2*Vtmanual;
    | Vh=yRecta1*Vhauto+yRecta2*Vhmanual;
    | 
    | end
  function y  = rectaDosPuntos(y2,y1,x2,x1,x,vm):
    | function y  = rectaDosPuntos(y2,y1,x2,x1,x,vm)
    | 
    | m=(y2-y1)/(x2-x1);
    | yRecta=m*(x-x1)+y1;
    | if(yRecta<0)
    |    yRecta=0; 
    | end
    | y=yRecta*vm;
    | end
  function yRecta =rectaDosPuntos(y2,y1,x2,x1,x):
    | function yRecta =rectaDosPuntos(y2,y1,x2,x1,x)
    | m=(y2-y1)/(x2-x1);
    | yRecta=m*(x-x1)+y1;
    | end

== matlab function ProyectoAutomatasSimulink_jona/Controlador/ControlTita/AjusteBordes ==
  data: distanciaSegMaxCarro input; distanciaSegMinCarro input; xt_max input; xt_min input; xt input; Vt input; Vtita output
function Vtita = fcn(distanciaSegMaxCarro,distanciaSegMinCarro,xt_max,xt_min,xt,Vt)

if  xt<distanciaSegMinCarro && Vt<0
    m=1/(distanciaSegMinCarro-xt_min);
    yRecta=m*(xt-xt_min);
    if yRecta<0
        yRecta=0;
    end
    Vt=yRecta*Vt;
elseif xt>distanciaSegMaxCarro &&Vt>0
    m=1/(distanciaSegMaxCarro-xt_max);
    yRecta=m*(xt-xt_max);
    if yRecta<0
        yRecta=0;
    end
    Vt=yRecta*Vt;
end
Vtita=Vt;

== matlab function ProyectoAutomatasSimulink_jona/Controlador/ControlTita/PIDangulo/CalculoGanancias ==
  data: Kisaa output; Ksaa output; baa output; lh input; ml input; Mti input; mci input; nai input
function [Kisaa,Ksaa,baa]= fcn(lh,ml,Mti,mci,nai)

persistent Mt
if isempty(Mt)
   Mt=Mti;
end
persistent mc
if isempty(mc)
   mc=mci;
end
persistent na
if isempty(na)
   na=nai;
end
persistent g
if isempty(g)
   g=9.80665;
end

Ma=(ml+Mt)/(mc+ml)*lh;
wa=(4*(Mt+ml)*Mt*g)/(2*(Mt+ml))*lh^-0.5;
wposa=10*wa;
baa=Ma*na*wposa;
Ksaa=baa*wposa;
Kisaa=Ksaa*wposa/na;
